simulink model "ControllerModeSelector_Harness"  (R2024a)
settings: configuration reference "csMultiInstance" (kept outside this file)
settings Model: DataDictionary=DD_ControllerModeSelector.sldd  Creator=The MathWorks, Inc.  LastModifiedBy=The MathWorks, Inc.
settings ConfigSetRef: SourceName=csMultiInstance

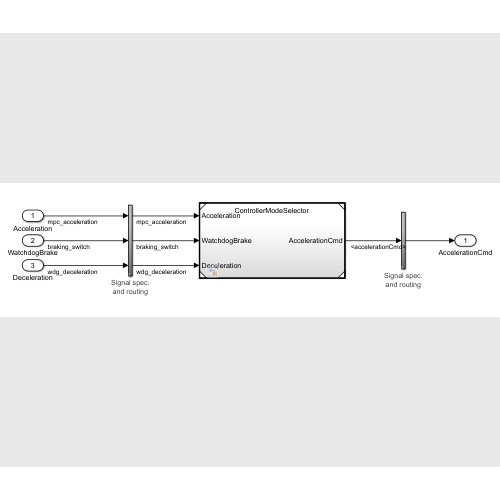
[thumbnail: Simulink's stored preview of the top-level diagram]
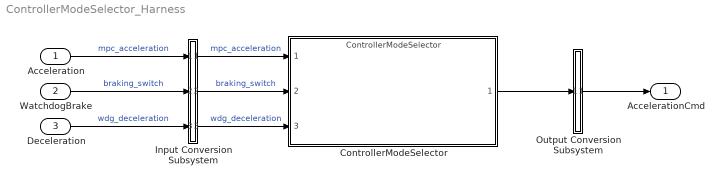
== system ControllerModeSelector_Harness ==
  Acceleration : Inport  OutDataTypeStr=double  PortDimensions=[1]  SampleTime=0.1
  WatchdogBrake : Inport  Port=2  OutDataTypeStr=Enum: BrStatus  PortDimensions=[1]  SampleTime=0.1  Interpolate=off
  Deceleration : Inport  Port=3  OutDataTypeStr=double  PortDimensions=[1]  SampleTime=0.1
  ControllerModeSelector : ModelReference  ModelNameDialog=ControllerModeSelector  SimulationMode=Normal  ModelReferenceVersion=7.0
  Input Conversion Subsystem : Subsystem  Tag=__SLT_ICS__  Description=|
      | Signal spec.
      | and routing
      settings: AttributesFormatString=%<Description>
  Output Conversion Subsystem : Subsystem  Tag=__SLT_OCS__  Description=|
      | Signal spec.
      | and routing
      settings: AttributesFormatString=%<Description>
  AccelerationCmd : Outport
  wires:
  Input Conversion Subsystem/1(Outport_1) -> ControllerModeSelector/1  "mpc_acceleration"
  WatchdogBrake/1 -> Input Conversion Subsystem/2(Inport_2)  "braking_switch"
  Output Conversion Subsystem/1(Outport_1) -> AccelerationCmd/1
  Input Conversion Subsystem/3(Outport_3) -> ControllerModeSelector/3  "wdg_deceleration"
  Deceleration/1 -> Input Conversion Subsystem/3(Inport_3)  "wdg_deceleration"
  Input Conversion Subsystem/2(Outport_2) -> ControllerModeSelector/2  "braking_switch"
  Acceleration/1 -> Input Conversion Subsystem/1(Inport_1)  "mpc_acceleration"
  ControllerModeSelector/1 -> Output Conversion Subsystem/1(Inport_1)

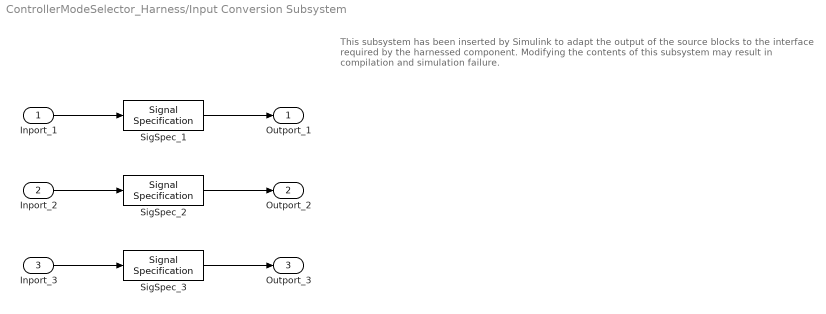
== system ControllerModeSelector_Harness/Input Conversion Subsystem ==
  note: This subsystem has been inserted by Simulink to adapt the output of the source blocks to the interface required by the harnessed component.
      |  Modifying the contents of this subsystem may result in compilation and simulation failure.
  Inport_1 : Inport
  Inport_2 : Inport  Port=2
  Inport_3 : Inport  Port=3
  SigSpec_1 : SignalSpecification  OutDataTypeStr=double  Unit=m/s^2  Dimensions=[1]  SampleTime=0.1
  SigSpec_2 : SignalSpecification  OutDataTypeStr=Enum: BrStatus  Dimensions=[1]  SampleTime=0.1
  SigSpec_3 : SignalSpecification  OutDataTypeStr=double  Unit=m/s^2  Dimensions=[1]  SampleTime=0.1
  Outport_1 : Outport
  Outport_2 : Outport  Port=2
  Outport_3 : Outport  Port=3
  wires:
  SigSpec_1/1 -> Outport_1/1
  Inport_1/1 -> SigSpec_1/1
  SigSpec_2/1 -> Outport_2/1
  Inport_2/1 -> SigSpec_2/1
  SigSpec_3/1 -> Outport_3/1
  Inport_3/1 -> SigSpec_3/1

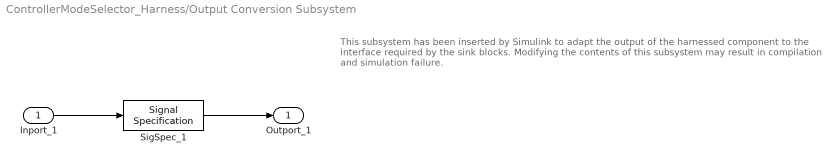
== system ControllerModeSelector_Harness/Output Conversion Subsystem ==
  note: This subsystem has been inserted by Simulink to adapt the output of the harnessed component to the interface required by the sink blocks.
      |  Modifying the contents of this subsystem may result in compilation and simulation failure.
  Inport_1 : Inport
  SigSpec_1 : SignalSpecification  OutDataTypeStr=double  Unit=m/s^2  Dimensions=[1]  SampleTime=0.1
  Outport_1 : Outport
  wires:
  Inport_1/1 -> SigSpec_1/1
  SigSpec_1/1 -> Outport_1/1
